simulink model "Tx_Rx"  (R2020a)
settings: Solver=VariableStepAuto  StartTime=0.0  StopTime=640e-9  RelTol=1e-3
libraries: msbUtilities x102, simulink_extras x15, dspswit3 x4, dspsigops x2
(part 2 of 3)

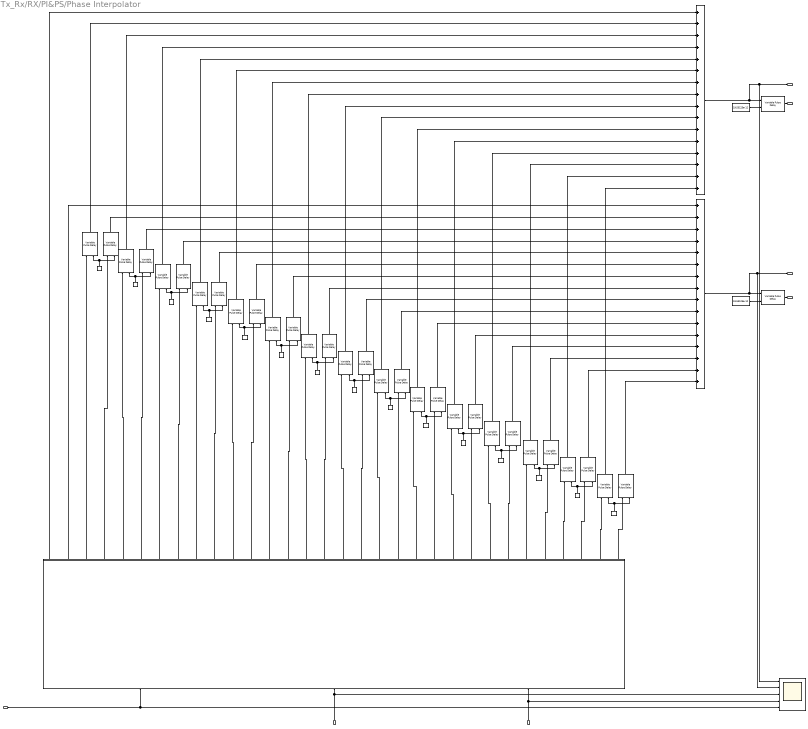
== system Tx_Rx/RX/PI&PS/Phase Interpolator ==
  CLK_s1 : Inport
  CLK_s3 : Inport  Port=2
  LSB_4bit : Inport  Port=3
  Add6 : Sum  Inputs=++++++++++++++++
  Add7 : Sum  Inputs=++++++++++++++++
  Constant26 : Constant  Value=19.53125e-12
  Constant27 : Constant  Value=0.6103515625e-12
  Constant28 : Constant  Value=2*0.6103515625e-12
  Constant29 : Constant  Value=3*0.6103515625e-12
  Constant30 : Constant  Value=4*0.6103515625e-12
  Constant31 : Constant  Value=5*0.6103515625e-12
  Constant32 : Constant  Value=6*0.6103515625e-12
  Constant33 : Constant  Value=7*0.6103515625e-12
  Constant34 : Constant  Value=8*0.6103515625e-12
  Constant35 : Constant  Value=9*0.6103515625e-12
  Constant36 : Constant  Value=10*0.6103515625e-12
  Constant37 : Constant  Value=11*0.6103515625e-12
  Constant38 : Constant  Value=12*0.6103515625e-12
  Constant39 : Constant  Value=13*0.6103515625e-12
  Constant40 : Constant  Value=14*0.6103515625e-12
  Constant41 : Constant  Value=15*0.6103515625e-12
  Constant42 : Constant  Value=19.53125e-12
  MATLAB Function : MATLAB Function  TreatAsAtomicUnit=on
  Scope : Scope  NumInputPorts=5
  Variable Pulse Delay{,1..31} (32 alike) : msbUtilities/Variable Pulse Delay  InitialInput=0  BufferSize=100
      settings: SourceProductBaseCode=AM
  CLK1 : Outport
  CLK2 : Outport  Port=2
  CLK3 : Outport  Port=3
  CLK4 : Outport  Port=4
  wires:
  Variable Pulse Delay30/1 -> Add6/16
  Constant40/1 -> Variable Pulse Delay28/2, Variable Pulse Delay29/2
  MATLAB Function/14(c6_1) -> Variable Pulse Delay13/1
  MATLAB Function/23(c11_0) -> Variable Pulse Delay22/1
  Constant34/1 -> Variable Pulse Delay17/2, Variable Pulse Delay16/2
  Constant41/1 -> Variable Pulse Delay31/2, Variable Pulse Delay30/2
  MATLAB Function/9(c4_0) -> Variable Pulse Delay8/1
  Variable Pulse Delay19/1 -> Add7/10
  Variable Pulse Delay6/1 -> Add6/4
  Constant35/1 -> Variable Pulse Delay19/2, Variable Pulse Delay18/2
  Constant27/1 -> Variable Pulse Delay2/2, Variable Pulse Delay3/2
  Variable Pulse Delay10/1 -> Add6/6
  Variable Pulse Delay25/1 -> Add7/13
  MATLAB Function/32(c15_1) -> Variable Pulse Delay31/1
  MATLAB Function/25(c12_0) -> Variable Pulse Delay24/1
  MATLAB Function/22(c10_1) -> Variable Pulse Delay21/1
  Constant33/1 -> Variable Pulse Delay15/2, Variable Pulse Delay14/2
  MATLAB Function/29(c14_0) -> Variable Pulse Delay28/1
  Constant36/1 -> Variable Pulse Delay21/2, Variable Pulse Delay20/2
  MATLAB Function/26(c12_1) -> Variable Pulse Delay25/1
  Variable Pulse Delay12/1 -> Add6/7
  Variable Pulse Delay22/1 -> Add6/12
  MATLAB Function/3(c1_0) -> Variable Pulse Delay2/1
  Constant28/1 -> Variable Pulse Delay5/2, Variable Pulse Delay4/2
  Constant31/1 -> Variable Pulse Delay11/2, Variable Pulse Delay10/2
  MATLAB Function/1(c0_0) -> Add6/1
  Constant30/1 -> Variable Pulse Delay9/2, Variable Pulse Delay8/2
  MATLAB Function/31(c15_0) -> Variable Pulse Delay30/1
  Constant38/1 -> Variable Pulse Delay25/2, Variable Pulse Delay24/2
  MATLAB Function/6(c2_1) -> Variable Pulse Delay5/1
  MATLAB Function/12(c5_1) -> Variable Pulse Delay11/1
  Variable Pulse Delay24/1 -> Add6/13
  Constant32/1 -> Variable Pulse Delay13/2, Variable Pulse Delay12/2
  MATLAB Function/17(c8_0) -> Variable Pulse Delay16/1
  MATLAB Function/15(c7_0) -> Variable Pulse Delay14/1
  Variable Pulse Delay8/1 -> Add6/5
  MATLAB Function/10(c4_1) -> Variable Pulse Delay9/1
  MATLAB Function/21(c10_0) -> Variable Pulse Delay20/1
  MATLAB Function/18(c8_1) -> Variable Pulse Delay17/1
  MATLAB Function/27(c13_0) -> Variable Pulse Delay26/1
  Variable Pulse Delay2/1 -> Add6/2
  Constant39/1 -> Variable Pulse Delay27/2, Variable Pulse Delay26/2
  MATLAB Function/2(c0_1) -> Add7/1
  Variable Pulse Delay16/1 -> Add6/9
  Variable Pulse Delay4/1 -> Add6/3
  Variable Pulse Delay18/1 -> Add6/10
  MATLAB Function/19(c9_0) -> Variable Pulse Delay18/1
  MATLAB Function/13(c6_0) -> Variable Pulse Delay12/1
  Variable Pulse Delay5/1 -> Add7/3
  Variable Pulse Delay17/1 -> Add7/9
  MATLAB Function/4(c1_1) -> Variable Pulse Delay3/1
  MATLAB Function/20(c9_1) -> Variable Pulse Delay19/1
  Variable Pulse Delay31/1 -> Add7/16
  Constant26/1 -> Variable Pulse Delay/2
  MATLAB Function/16(c7_1) -> Variable Pulse Delay15/1
  Constant42/1 -> Variable Pulse Delay1/2
  Variable Pulse Delay27/1 -> Add7/14
  Add6/1 -> CLK1/1, Scope/1, Variable Pulse Delay/1
  Variable Pulse Delay26/1 -> Add6/14
  Constant29/1 -> Variable Pulse Delay7/2, Variable Pulse Delay6/2
  Variable Pulse Delay13/1 -> Add7/7
  Variable Pulse Delay14/1 -> Add6/8
  Variable Pulse Delay29/1 -> Add7/15
  Variable Pulse Delay28/1 -> Add6/15
  MATLAB Function/28(c13_1) -> Variable Pulse Delay27/1
  Variable Pulse Delay3/1 -> Add7/2
  MATLAB Function/24(c11_1) -> Variable Pulse Delay23/1
  MATLAB Function/11(c5_0) -> Variable Pulse Delay10/1
  Variable Pulse Delay7/1 -> Add7/4
  MATLAB Function/5(c2_0) -> Variable Pulse Delay4/1
  Constant37/1 -> Variable Pulse Delay23/2, Variable Pulse Delay22/2
  MATLAB Function/30(c14_1) -> Variable Pulse Delay29/1
  Variable Pulse Delay21/1 -> Add7/11
  Variable Pulse Delay15/1 -> Add7/8
  Variable Pulse Delay20/1 -> Add6/11
  Variable Pulse Delay9/1 -> Add7/5
  Variable Pulse Delay11/1 -> Add7/6
  MATLAB Function/7(c3_0) -> Variable Pulse Delay6/1
  MATLAB Function/8(c3_1) -> Variable Pulse Delay7/1
  Variable Pulse Delay23/1 -> Add7/12
  Add7/1 -> CLK3/1, Scope/2, Variable Pulse Delay1/1
  LSB_4bit/1 -> MATLAB Function/1(LSB_4bit), Scope/5
  Variable Pulse Delay/1 -> CLK2/1
  Variable Pulse Delay1/1 -> CLK4/1
  CLK_s1/1 -> MATLAB Function/2(clk_s1), Scope/3
  CLK_s3/1 -> MATLAB Function/3(clk_s3), Scope/4

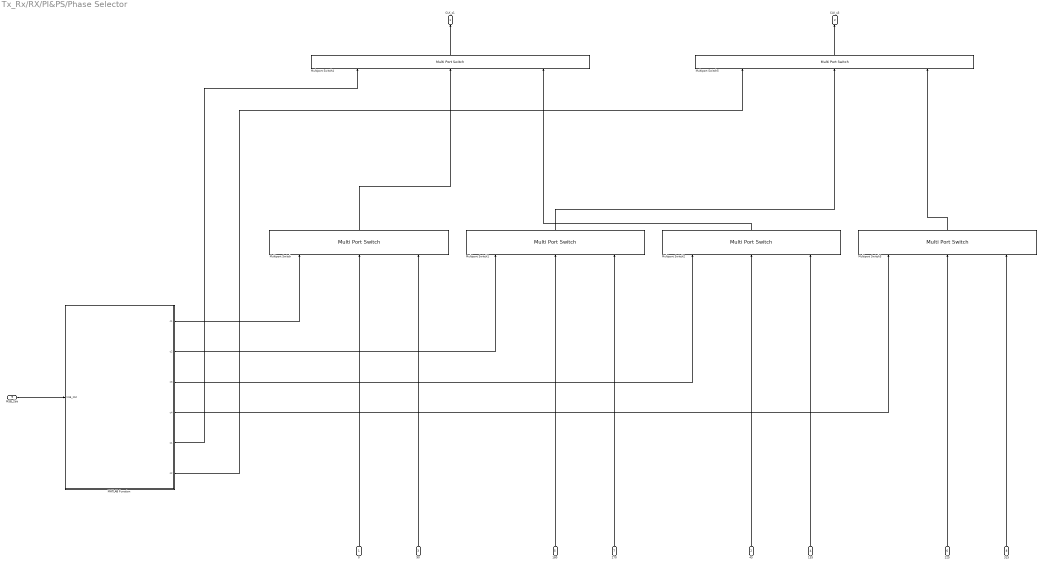
== system Tx_Rx/RX/PI&PS/Phase Selector ==
  0 : Inport
  45 : Inport  Port=2
  90 : Inport  Port=3
  135 : Inport  Port=4
  180 : Inport  Port=5
  225 : Inport  Port=6
  270 : Inport  Port=7
  315 : Inport  Port=8
  MSB_2bit : Inport  Port=9
  MATLAB Function : MATLAB Function  TreatAsAtomicUnit=on
  Multiport Switch{,1..5} (6 alike) : MultiPortSwitch  Inputs=2
  CLK_s1 : Outport
  CLK_s3 : Outport  Port=2
  wires:
  Multiport Switch1/1 -> Multiport Switch5/2
  Multiport Switch2/1 -> Multiport Switch4/3
  Multiport Switch/1 -> Multiport Switch4/2
  Multiport Switch3/1 -> Multiport Switch5/3
  225/1 -> Multiport Switch3/2
  135/1 -> Multiport Switch2/3
  0/1 -> Multiport Switch/2
  45/1 -> Multiport Switch2/2
  90/1 -> Multiport Switch/3
  315/1 -> Multiport Switch3/3
  270/1 -> Multiport Switch1/3
  180/1 -> Multiport Switch1/2
  Multiport Switch5/1 -> CLK_s3/1
  Multiport Switch4/1 -> CLK_s1/1
  MSB_2bit/1 -> MATLAB Function/1(MSB_2bit)
  MATLAB Function/1(c1) -> Multiport Switch/1
  MATLAB Function/2(c2) -> Multiport Switch1/1
  MATLAB Function/3(c3) -> Multiport Switch2/1
  MATLAB Function/4(c4) -> Multiport Switch3/1
  MATLAB Function/5(s1) -> Multiport Switch4/1
  MATLAB Function/6(s2) -> Multiport Switch5/1

== system Tx_Rx/TX/Delay Line1/Subsystem32 ==
  N-1 : Inport
  Constant : Constant
  Divide : Product  Inputs=*/
  Fref : Gain  Gain=78.125e-12
  Num : Gain  Gain=8
  Relay1 : Relay
  Variable Time Delay : VariableTransportDelay  MaximumDelay=10  FixedBuffer=on
  N : Outport
  wires:
  Num/1 -> Divide/2
  N-1/1 -> Variable Time Delay/1
  Relay1/1 -> N/1
  Divide/1 -> Fref/1
  Fref/1 -> Variable Time Delay/2
  Variable Time Delay/1 -> Relay1/1
  Constant/1 -> Num/1, Divide/1

== system Tx_Rx/TX/Delay Line1/Subsystem33 ==
  N-1 : Inport
  Constant : Constant
  Divide : Product  Inputs=*/
  Fref : Gain  Gain=78.125e-12
  Num : Gain  Gain=8
  Relay1 : Relay
  Variable Time Delay : VariableTransportDelay  MaximumDelay=10  FixedBuffer=on
  N : Outport
  wires:
  Num/1 -> Divide/2
  N-1/1 -> Variable Time Delay/1
  Relay1/1 -> N/1
  Divide/1 -> Fref/1
  Fref/1 -> Variable Time Delay/2
  Variable Time Delay/1 -> Relay1/1
  Constant/1 -> Num/1, Divide/1

== system Tx_Rx/TX/Delay Line1/Subsystem34 ==
  N-1 : Inport
  Constant : Constant
  Divide : Product  Inputs=*/
  Fref : Gain  Gain=78.125e-12
  Num : Gain  Gain=8
  Relay1 : Relay
  Variable Time Delay : VariableTransportDelay  MaximumDelay=10  FixedBuffer=on
  N : Outport
  wires:
  Num/1 -> Divide/2
  N-1/1 -> Variable Time Delay/1
  Relay1/1 -> N/1
  Divide/1 -> Fref/1
  Fref/1 -> Variable Time Delay/2
  Variable Time Delay/1 -> Relay1/1
  Constant/1 -> Num/1, Divide/1

== system Tx_Rx/TX/Delay Line1/Subsystem35 ==
  N-1 : Inport
  Constant : Constant
  Divide : Product  Inputs=*/
  Fref : Gain  Gain=78.125e-12
  Num : Gain  Gain=8
  Relay1 : Relay
  Variable Time Delay : VariableTransportDelay  MaximumDelay=10  FixedBuffer=on
  N : Outport
  wires:
  Num/1 -> Divide/2
  N-1/1 -> Variable Time Delay/1
  Relay1/1 -> N/1
  Divide/1 -> Fref/1
  Fref/1 -> Variable Time Delay/2
  Variable Time Delay/1 -> Relay1/1
  Constant/1 -> Num/1, Divide/1

== system Tx_Rx/TX/Delay Line1/Subsystem36 ==
  N-1 : Inport
  Constant : Constant
  Divide : Product  Inputs=*/
  Fref : Gain  Gain=78.125e-12
  Num : Gain  Gain=8
  Relay1 : Relay
  Variable Time Delay : VariableTransportDelay  MaximumDelay=10  FixedBuffer=on
  N : Outport
  wires:
  Num/1 -> Divide/2
  N-1/1 -> Variable Time Delay/1
  Relay1/1 -> N/1
  Divide/1 -> Fref/1
  Fref/1 -> Variable Time Delay/2
  Variable Time Delay/1 -> Relay1/1
  Constant/1 -> Num/1, Divide/1

== system Tx_Rx/TX/Delay Line1/Subsystem37 ==
  N-1 : Inport
  Constant : Constant
  Divide : Product  Inputs=*/
  Fref : Gain  Gain=78.125e-12
  Num : Gain  Gain=8
  Relay1 : Relay
  Variable Time Delay : VariableTransportDelay  MaximumDelay=10  FixedBuffer=on
  N : Outport
  wires:
  Num/1 -> Divide/2
  N-1/1 -> Variable Time Delay/1
  Relay1/1 -> N/1
  Divide/1 -> Fref/1
  Fref/1 -> Variable Time Delay/2
  Variable Time Delay/1 -> Relay1/1
  Constant/1 -> Num/1, Divide/1

== system Tx_Rx/TX/Delay Line1/Subsystem38 ==
  N-1 : Inport
  Constant : Constant
  Divide : Product  Inputs=*/
  Fref : Gain  Gain=78.125e-12
  Num : Gain  Gain=8
  Relay1 : Relay
  Variable Time Delay : VariableTransportDelay  MaximumDelay=10  FixedBuffer=on
  N : Outport
  wires:
  Num/1 -> Divide/2
  N-1/1 -> Variable Time Delay/1
  Relay1/1 -> N/1
  Divide/1 -> Fref/1
  Fref/1 -> Variable Time Delay/2
  Variable Time Delay/1 -> Relay1/1
  Constant/1 -> Num/1, Divide/1

== system Tx_Rx/TX/Delay Line1/Subsystem39 ==
  N-1 : Inport
  Constant : Constant
  Divide : Product  Inputs=*/
  Fref : Gain  Gain=78.125e-12
  Num : Gain  Gain=8
  Relay1 : Relay
  Variable Time Delay : VariableTransportDelay  MaximumDelay=10  FixedBuffer=on
  N : Outport
  wires:
  Num/1 -> Divide/2
  N-1/1 -> Variable Time Delay/1
  Relay1/1 -> N/1
  Divide/1 -> Fref/1
  Fref/1 -> Variable Time Delay/2
  Variable Time Delay/1 -> Relay1/1
  Constant/1 -> Num/1, Divide/1

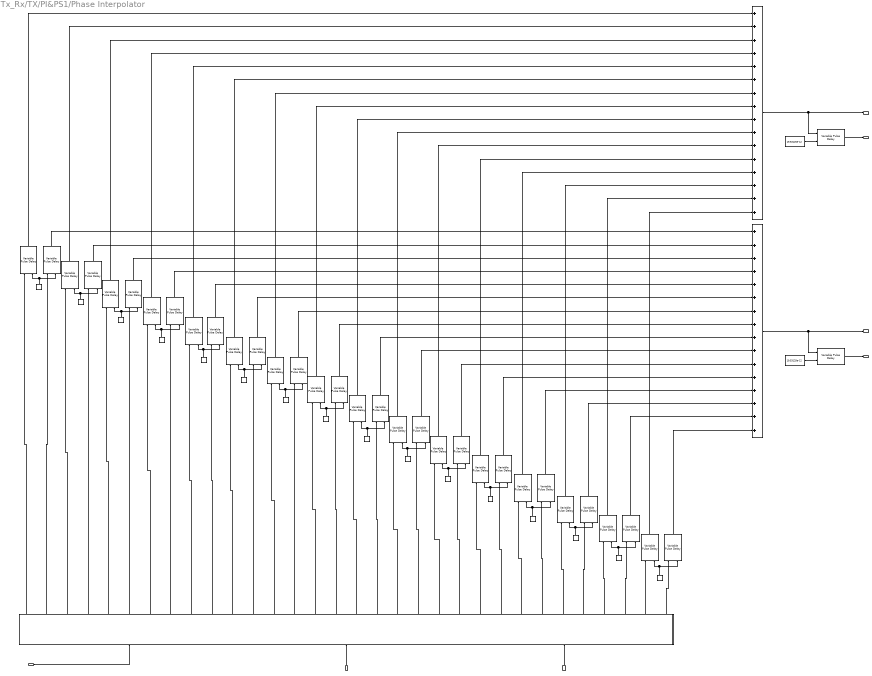
== system Tx_Rx/TX/PI&PS1/Phase Interpolator ==
  CLK_s1 : Inport
  CLK_s3 : Inport  Port=2
  LSB_4bit : Inport  Port=3
  Add6 : Sum  Inputs=++++++++++++++++
  Add7 : Sum  Inputs=++++++++++++++++
  Constant1 : Constant  Value=16*0.6103515625e-12
  Constant2 : Constant  Value=19.53125e-12
  Constant26 : Constant  Value=19.53125e-12
  Constant27 : Constant  Value=0.6103515625e-12
  Constant28 : Constant  Value=2*0.6103515625e-12
  Constant29 : Constant  Value=3*0.6103515625e-12
  Constant30 : Constant  Value=4*0.6103515625e-12
  Constant31 : Constant  Value=5*0.6103515625e-12
  Constant32 : Constant  Value=6*0.6103515625e-12
  Constant33 : Constant  Value=7*0.6103515625e-12
  Constant34 : Constant  Value=8*0.6103515625e-12
  Constant35 : Constant  Value=9*0.6103515625e-12
  Constant36 : Constant  Value=10*0.6103515625e-12
  Constant37 : Constant  Value=11*0.6103515625e-12
  Constant38 : Constant  Value=12*0.6103515625e-12
  Constant39 : Constant  Value=13*0.6103515625e-12
  Constant40 : Constant  Value=14*0.6103515625e-12
  Constant41 : Constant  Value=15*0.6103515625e-12
  MATLAB Function : MATLAB Function  TreatAsAtomicUnit=on
  Variable Pulse Delay{,1..33} (34 alike) : msbUtilities/Variable Pulse Delay  InitialInput=0  BufferSize=100
      settings: SourceProductBaseCode=AM
  CLK1 : Outport
  CLK3 : Outport  Port=2
  CLK2 : Outport  Port=3
  CLK4 : Outport  Port=4
  wires:
  Variable Pulse Delay30/1 -> Add6/16
  Constant40/1 -> Variable Pulse Delay28/2, Variable Pulse Delay29/2
  MATLAB Function/14(c6_1) -> Variable Pulse Delay13/1
  MATLAB Function/23(c11_0) -> Variable Pulse Delay22/1
  Constant34/1 -> Variable Pulse Delay17/2, Variable Pulse Delay16/2
  Constant41/1 -> Variable Pulse Delay31/2, Variable Pulse Delay30/2
  MATLAB Function/9(c4_0) -> Variable Pulse Delay8/1
  Variable Pulse Delay19/1 -> Add7/10
  Variable Pulse Delay6/1 -> Add6/4
  Constant35/1 -> Variable Pulse Delay19/2, Variable Pulse Delay18/2
  Constant27/1 -> Variable Pulse Delay2/2, Variable Pulse Delay3/2
  Variable Pulse Delay10/1 -> Add6/6
  Variable Pulse Delay25/1 -> Add7/13
  MATLAB Function/32(c15_1) -> Variable Pulse Delay31/1
  MATLAB Function/25(c12_0) -> Variable Pulse Delay24/1
  MATLAB Function/22(c10_1) -> Variable Pulse Delay21/1
  Constant33/1 -> Variable Pulse Delay15/2, Variable Pulse Delay14/2
  MATLAB Function/29(c14_0) -> Variable Pulse Delay28/1
  Constant36/1 -> Variable Pulse Delay21/2, Variable Pulse Delay20/2
  MATLAB Function/26(c12_1) -> Variable Pulse Delay25/1
  Variable Pulse Delay12/1 -> Add6/7
  Variable Pulse Delay22/1 -> Add6/12
  MATLAB Function/3(c1_0) -> Variable Pulse Delay2/1
  Constant28/1 -> Variable Pulse Delay5/2, Variable Pulse Delay4/2
  Constant31/1 -> Variable Pulse Delay11/2, Variable Pulse Delay10/2
  Constant30/1 -> Variable Pulse Delay9/2, Variable Pulse Delay8/2
  MATLAB Function/31(c15_0) -> Variable Pulse Delay30/1
  Constant38/1 -> Variable Pulse Delay25/2, Variable Pulse Delay24/2
  MATLAB Function/6(c2_1) -> Variable Pulse Delay5/1
  MATLAB Function/12(c5_1) -> Variable Pulse Delay11/1
  Variable Pulse Delay24/1 -> Add6/13
  Constant32/1 -> Variable Pulse Delay13/2, Variable Pulse Delay12/2
  MATLAB Function/17(c8_0) -> Variable Pulse Delay16/1
  MATLAB Function/15(c7_0) -> Variable Pulse Delay14/1
  Variable Pulse Delay8/1 -> Add6/5
  MATLAB Function/10(c4_1) -> Variable Pulse Delay9/1
  MATLAB Function/21(c10_0) -> Variable Pulse Delay20/1
  MATLAB Function/18(c8_1) -> Variable Pulse Delay17/1
  MATLAB Function/27(c13_0) -> Variable Pulse Delay26/1
  Variable Pulse Delay2/1 -> Add6/2
  Constant39/1 -> Variable Pulse Delay27/2, Variable Pulse Delay26/2
  Variable Pulse Delay16/1 -> Add6/9
  Variable Pulse Delay4/1 -> Add6/3
  Variable Pulse Delay18/1 -> Add6/10
  MATLAB Function/19(c9_0) -> Variable Pulse Delay18/1
  MATLAB Function/13(c6_0) -> Variable Pulse Delay12/1
  Variable Pulse Delay5/1 -> Add7/3
  Variable Pulse Delay17/1 -> Add7/9
  MATLAB Function/4(c1_1) -> Variable Pulse Delay3/1
  MATLAB Function/20(c9_1) -> Variable Pulse Delay19/1
  Variable Pulse Delay31/1 -> Add7/16
  MATLAB Function/16(c7_1) -> Variable Pulse Delay15/1
  Variable Pulse Delay27/1 -> Add7/14
  Variable Pulse Delay26/1 -> Add6/14
  Constant29/1 -> Variable Pulse Delay7/2, Variable Pulse Delay6/2
  Variable Pulse Delay13/1 -> Add7/7
  Variable Pulse Delay14/1 -> Add6/8
  Variable Pulse Delay29/1 -> Add7/15
  Variable Pulse Delay28/1 -> Add6/15
  MATLAB Function/28(c13_1) -> Variable Pulse Delay27/1
  Variable Pulse Delay3/1 -> Add7/2
  MATLAB Function/24(c11_1) -> Variable Pulse Delay23/1
  MATLAB Function/11(c5_0) -> Variable Pulse Delay10/1
  Variable Pulse Delay7/1 -> Add7/4
  MATLAB Function/5(c2_0) -> Variable Pulse Delay4/1
  Constant37/1 -> Variable Pulse Delay23/2, Variable Pulse Delay22/2
  MATLAB Function/30(c14_1) -> Variable Pulse Delay29/1
  Variable Pulse Delay21/1 -> Add7/11
  Variable Pulse Delay15/1 -> Add7/8
  Variable Pulse Delay20/1 -> Add6/11
  Variable Pulse Delay9/1 -> Add7/5
  Variable Pulse Delay11/1 -> Add7/6
  MATLAB Function/7(c3_0) -> Variable Pulse Delay6/1
  MATLAB Function/8(c3_1) -> Variable Pulse Delay7/1
  Variable Pulse Delay23/1 -> Add7/12
  LSB_4bit/1 -> MATLAB Function/1(LSB_4bit)
  Add6/1 -> Variable Pulse Delay/1, CLK1/1
  CLK_s1/1 -> MATLAB Function/2(clk_s1)
  CLK_s3/1 -> MATLAB Function/3(clk_s3)
  MATLAB Function/1(c0_0) -> Variable Pulse Delay1/1
  MATLAB Function/2(c0_1) -> Variable Pulse Delay32/1
  Variable Pulse Delay1/1 -> Add6/1
  Variable Pulse Delay32/1 -> Add7/1
  Constant1/1 -> Variable Pulse Delay32/2, Variable Pulse Delay1/2
  Variable Pulse Delay/1 -> CLK2/1
  Constant26/1 -> Variable Pulse Delay/2
  Variable Pulse Delay33/1 -> CLK4/1
  Add7/1 -> Variable Pulse Delay33/1, CLK3/1
  Constant2/1 -> Variable Pulse Delay33/2

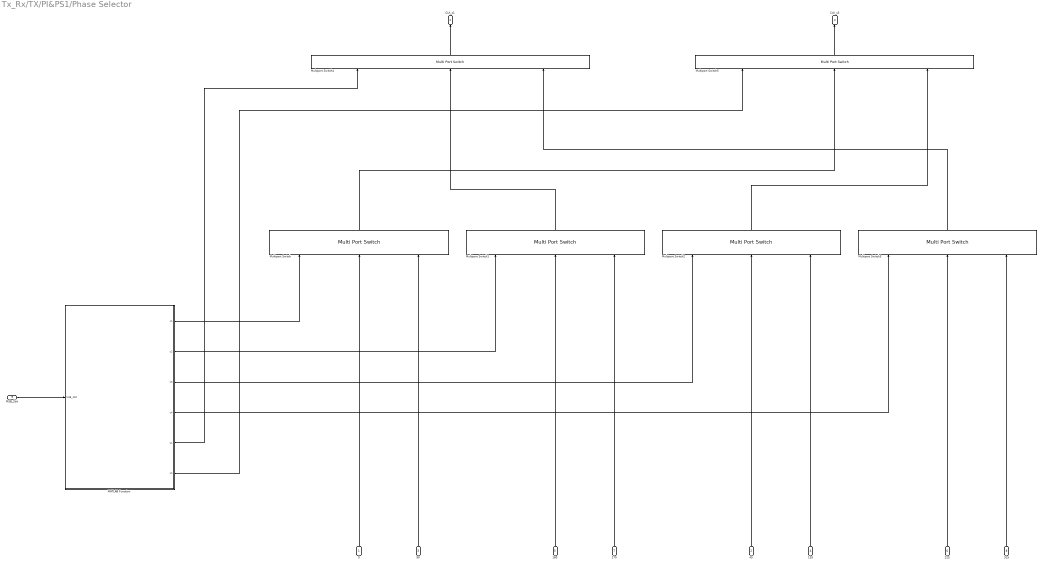
== system Tx_Rx/TX/PI&PS1/Phase Selector ==
  0 : Inport
  45 : Inport  Port=2
  90 : Inport  Port=3
  135 : Inport  Port=4
  180 : Inport  Port=5
  225 : Inport  Port=6
  270 : Inport  Port=7
  315 : Inport  Port=8
  MSB_2bit : Inport  Port=9
  MATLAB Function : MATLAB Function  TreatAsAtomicUnit=on
  Multiport Switch{,1..5} (6 alike) : MultiPortSwitch  Inputs=2
  CLK_s1 : Outport
  CLK_s3 : Outport  Port=2
  wires:
  225/1 -> Multiport Switch3/2
  135/1 -> Multiport Switch2/3
  0/1 -> Multiport Switch/2
  45/1 -> Multiport Switch2/2
  90/1 -> Multiport Switch/3
  315/1 -> Multiport Switch3/3
  270/1 -> Multiport Switch1/3
  180/1 -> Multiport Switch1/2
  Multiport Switch5/1 -> CLK_s3/1
  Multiport Switch4/1 -> CLK_s1/1
  MSB_2bit/1 -> MATLAB Function/1(MSB_2bit)
  MATLAB Function/1(c1) -> Multiport Switch/1
  MATLAB Function/2(c2) -> Multiport Switch1/1
  MATLAB Function/3(c3) -> Multiport Switch2/1
  MATLAB Function/4(c4) -> Multiport Switch3/1
  MATLAB Function/5(s1) -> Multiport Switch4/1
  MATLAB Function/6(s2) -> Multiport Switch5/1
  Multiport Switch/1 -> Multiport Switch5/2
  Multiport Switch2/1 -> Multiport Switch5/3
  Multiport Switch1/1 -> Multiport Switch4/2
  Multiport Switch3/1 -> Multiport Switch4/3

== matlab function Tx_Rx/BER_calculator/PI&PS/Phase Selector/MATLAB Function ==
  data: MSB_2bit input; c1 output; c2 output; c3 output; c4 output; s1 output; s2 output
function [c1,c2,c3,c4,s1,s2] =  bit_decoder(MSB_2bit)
    if (MSB_2bit == 0)
        c1 = 1;
        c2 = 1;
        c3 = 1;
        c4 = 1;
        s1 = 1;
        s2 = 1;
    elseif (MSB_2bit == 1)
        c1 = 2;
        c2 = 2;
        c3 = 1;
        c4 = 1;
        s1 = 2;
        s2 = 2;
    elseif (MSB_2bit == 10)
        c1 = 2;
        c2 = 2;
        c3 = 2;
        c4 = 2;
        s1 = 1;
        s2 = 1;
    elseif (MSB_2bit == 11)
        c1 = 1;
        c2 = 1;
        c3 = 2;
        c4 = 2;
        s1 = 2;
        s2 = 2;
    else
        c1 = 1;
        c2 = 1;
        c3 = 1;
        c4 = 1;
        s1 = 1;
        s2 = 1;
    end

== matlab function Tx_Rx/TX/MATLAB Function ==
  data: data_in_ref input; data_in_change input; LSB_4bit input; data_out output; MSB_2bit input
function data_out  = bypass_000000(data_in_ref,data_in_change,LSB_4bit,MSB_2bit)
    if(LSB_4bit == 0000&&MSB_2bit == 00)
        data_out = data_in_ref;
    else
        data_out = data_in_change;
    end
end

== matlab function Tx_Rx/TX/PI&PS1/Phase Interpolator/MATLAB Function ==
  data: LSB_4bit input; c0_0 output; clk_s1 input; clk_s3 input; c0_1 output; c1_0 output; c1_1 output; c2_0 output; c2_1 output; c3_0 output; c3_1 output; c4_0 output; c4_1 output; c5_0 output; c5_1 output; c6_0 output; c6_1 output; c7_0 output; c7_1 output; c8_0 output; c8_1 output; c9_0 output; c9_1 output; c10_0 output; c10_1 output; c11_0 output; c11_1 output; c12_0 output; c12_1 output; c13_0 output; c13_1 output; c14_0 output; c14_1 output; c15_0 output; c15_1 output
function [c0_0,c0_1,c1_0,c1_1,c2_0,c2_1,c3_0,c3_1,c4_0,c4_1,c5_0,c5_1,c6_0,c6_1,c7_0,c7_1,c8_0,c8_1,c9_0,c9_1,c10_0,c10_1,c11_0,c11_1,c12_0,c12_1,c13_0,c13_1,c14_0,c14_1,c15_0,c15_1] = phase_interpolator(LSB_4bit,clk_s1,clk_s3)
    switch LSB_4bit
        case 0
            c0_0 = clk_s1;
            c0_1 = clk_s3;
            c1_0 = 0;
            c1_1 = 0;
            c2_0 = 0;
            c2_1 = 0;
            c3_0 = 0;
            c3_1 = 0;
            c4_0 = 0;
            c4_1 = 0;
            c5_0 = 0;
            c5_1 = 0;
            c6_0 = 0;
            c6_1 = 0;
            c7_0 = 0;
            c7_1 = 0;
            c8_0 = 0;
            c8_1 = 0;
            c9_0 = 0;
            c9_1 = 0;
            c10_0 = 0;
            c10_1 = 0;
            c11_0 = 0;
            c11_1 = 0;
            c12_0 = 0;
            c12_1 = 0;
            c13_0 = 0;
            c13_1 = 0;
            c14_0 = 0;
            c14_1 = 0;
            c15_0 = 0;
            c15_1 = 0;
        case 1111
            c0_0 = 0;
            c0_1 = 0;
            c1_0 = clk_s1;
            c1_1 = clk_s3;
            c2_0 = 0;
            c2_1 = 0;
            c3_0 = 0;
            c3_1 = 0;
            c4_0 = 0;
            c4_1 = 0;
            c5_0 = 0;
            c5_1 = 0;
            c6_0 = 0;
            c6_1 = 0;
            c7_0 = 0;
            c7_1 = 0;
            c8_0 = 0;
            c8_1 = 0;
            c9_0 = 0;
            c9_1 = 0;
            c10_0 = 0;
            c10_1 = 0;
            c11_0 = 0;
            c11_1 = 0;
            c12_0 = 0;
            c12_1 = 0;
            c13_0 = 0;
            c13_1 = 0;
            c14_0 = 0;
            c14_1 = 0;
            c15_0 = 0;
            c15_1 = 0;
        case 1110
            c0_0 = 0;
            c0_1 = 0;
            c1_0 = 0;
            c1_1 = 0;
            c2_0 = clk_s1;
            c2_1 = clk_s3;
            c3_0 = 0;
            c3_1 = 0;
            c4_0 = 0;
            c4_1 = 0;
            c5_0 = 0;
            c5_1 = 0;
            c6_0 = 0;
            c6_1 = 0;
            c7_0 = 0;
            c7_1 = 0;
            c8_0 = 0;
            c8_1 = 0;
            c9_0 = 0;
            c9_1 = 0;
            c10_0 = 0;
            c10_1 = 0;
            c11_0 = 0;
            c11_1 = 0;
            c12_0 = 0;
            c12_1 = 0;
            c13_0 = 0;
            c13_1 = 0;
            c14_0 = 0;
            c14_1 = 0;
            c15_0 = 0;
            c15_1 = 0;
        case 1101
            c0_0 = 0;
            c0_1 = 0;
            c1_0 = 0;
            c1_1 = 0;
            c2_0 = 0;
            c2_1 = 0;
            c3_0 = clk_s1;
            c3_1 = clk_s3;
            c4_0 = 0;
            c4_1 = 0;
            c5_0 = 0;
            c5_1 = 0;
            c6_0 = 0;
            c6_1 = 0;
            c7_0 = 0;
            c7_1 = 0;
            c8_0 = 0;
            c8_1 = 0;
            c9_0 = 0;
            c9_1 = 0;
            c10_0 = 0;
            c10_1 = 0;
            c11_0 = 0;
            c11_1 = 0;
            c12_0 = 0;
            c12_1 = 0;
            c13_0 = 0;
            c13_1 = 0;
            c14_0 = 0;
            c14_1 = 0;
            c15_0 = 0;
            c15_1 = 0;
        case 1100
            c0_0 = 0;
            c0_1 = 0;
            c1_0 = 0;
            c1_1 = 0;
            c2_0 = 0;
            c2_1 = 0;
            c3_0 = 0;
            c3_1 = 0;
            c4_0 = clk_s1;
            c4_1 = clk_s3;
            c5_0 = 0;
            c5_1 = 0;
            c6_0 = 0;
            c6_1 = 0;
            c7_0 = 0;
            c7_1 = 0;
            c8_0 = 0;
            c8_1 = 0;
            c9_0 = 0;
            c9_1 = 0;
            c10_0 = 0;
            c10_1 = 0;
            c11_0 = 0;
            c11_1 = 0;
            c12_0 = 0;
            c12_1 = 0;
            c13_0 = 0;
            c13_1 = 0;
            c14_0 = 0;
            c14_1 = 0;
            c15_0 = 0;
            c15_1 = 0;
        case 1011
            c0_0 = 0;
            c0_1 = 0;
            c1_0 = 0;
            c1_1 = 0;
            c2_0 = 0;
            c2_1 = 0;
            c3_0 = 0;
            c3_1 = 0;
            c4_0 = 0;
            c4_1 = 0;
            c5_0 = clk_s1;
            c5_1 = clk_s3;
            c6_0 = 0;
            c6_1 = 0;
            c7_0 = 0;
            c7_1 = 0;
            c8_0 = 0;
            c8_1 = 0;
            c9_0 = 0;
            c9_1 = 0;
            c10_0 = 0;
            c10_1 = 0;
            c11_0 = 0;
            c11_1 = 0;
            c12_0 = 0;
            c12_1 = 0;
            c13_0 = 0;
            c13_1 = 0;
            c14_0 = 0;
            c14_1 = 0;
            c15_0 = 0;
            c15_1 = 0;
        case 1010
            c0_0 = 0;
            c0_1 = 0;
            c1_0 = 0;
            c1_1 = 0;
            c2_0 = 0;
            c2_1 = 0;
            c3_0 = 0;
            c3_1 = 0;
            c4_0 = 0;
            c4_1 = 0;
            c5_0 = 0;
            c5_1 = 0;
            c6_0 = clk_s1;
            c6_1 = clk_s3;
            c7_0 = 0;
            c7_1 = 0;
            c8_0 = 0;
            c8_1 = 0;
            c9_0 = 0;
            c9_1 = 0;
            c10_0 = 0;
            c10_1 = 0;
            c11_0 = 0;
            c11_1 = 0;
            c12_0 = 0;
            c12_1 = 0;
            c13_0 = 0;
            c13_1 = 0;
            c14_0 = 0;
            c14_1 = 0;
            c15_0 = 0;
            c15_1 = 0;
        case 1001
            c0_0 = 0;
            c0_1 = 0;
            c1_0 = 0;
            c1_1 = 0;
            c2_0 = 0;
            c2_1 = 0;
            c3_0 = 0;
            c3_1 = 0;
            c4_0 = 0;
            c4_1 = 0;
            c5_0 = 0;
            c5_1 = 0;
            c6_0 = 0;
            c6_1 = 0;
            c7_0 = clk_s1;
            c7_1 = clk_s3;
            c8_0 = 0;
            c8_1 = 0;
            c9_0 = 0;
            c9_1 = 0;
            c10_0 = 0;
            c10_1 = 0;
            c11_0 = 0;
            c11_1 = 0;
            c12_0 = 0;
            c12_1 = 0;
            c13_0 = 0;
            c13_1 = 0;
            c14_0 = 0;
            c14_1 = 0;
            c15_0 = 0;
            c15_1 = 0;
        case 1000
            c0_0 = 0;
            c0_1 = 0;
            c1_0 = 0;
            c1_1 = 0;
            c2_0 = 0;
            c2_1 = 0;
            c3_0 = 0;
            c3_1 = 0;
            c4_0 = 0;
            c4_1 = 0;
            c5_0 = 0;
            c5_1 = 0;
            c6_0 = 0;
            c6_1 = 0;
            c7_0 = 0;
            c7_1 = 0;
            c8_0 = clk_s1;
            c8_1 = clk_s3;
            c9_0 = 0;
            c9_1 = 0;
            c10_0 = 0;
            c10_1 = 0;
            c11_0 = 0;
            c11_1 = 0;
            c12_0 = 0;
            c12_1 = 0;
            c13_0 = 0;
            c13_1 = 0;
            c14_0 = 0;
            c14_1 = 0;
            c15_0 = 0;
            c15_1 = 0;
        case 111
            c0_0 = 0;
            c0_1 = 0;
            c1_0 = 0;
            c1_1 = 0;
            c2_0 = 0;
            c2_1 = 0;
            c3_0 = 0;
            c3_1 = 0;
            c4_0 = 0;
            c4_1 = 0;
            c5_0 = 0;
            c5_1 = 0;
            c6_0 = 0;
            c6_1 = 0;
            c7_0 = 0;
            c7_1 = 0;
            c8_0 = 0;
            c8_1 = 0;
            c9_0 = clk_s1;
            c9_1 = clk_s3;
            c10_0 = 0;
            c10_1 = 0;
            c11_0 = 0;
            c11_1 = 0;
            c12_0 = 0;
            c12_1 = 0;
            c13_0 = 0;
            c13_1 = 0;
            c14_0 = 0;
            c14_1 = 0;
            c15_0 = 0;
            c15_1 = 0;
        case 110
            c0_0 = 0;
            c0_1 = 0;
            c1_0 = 0;
            c1_1 = 0;
            c2_0 = 0;
            c2_1 = 0;
            c3_0 = 0;
            c3_1 = 0;
            c4_0 = 0;
            c4_1 = 0;
            c5_0 = 0;
            c5_1 = 0;
            c6_0 = 0;
            c6_1 = 0;
            c7_0 = 0;
            c7_1 = 0;
            c8_0 = 0;
            c8_1 = 0;
            c9_0 = 0;
            c9_1 = 0;
            c10_0 = clk_s1;
            c10_1 = clk_s3;
            c11_0 = 0;
            c11_1 = 0;
            c12_0 = 0;
            c12_1 = 0;
            c13_0 = 0;
            c13_1 = 0;
            c14_0 = 0;
            c14_1 = 0;
            c15_0 = 0;
            c15_1 = 0;   
        case 101
            c0_0 = 0;
            c0_1 = 0;
            c1_0 = 0;
            c1_1 = 0;
            c2_0 = 0;
            c2_1 = 0;
            c3_0 = 0;
            c3_1 = 0;
            c4_0 = 0;
            c4_1 = 0;
            c5_0 = 0;
            c5_1 = 0;
            c6_0 = 0;
            c6_1 = 0;
            c7_0 = 0;
            c7_1 = 0;
            c8_0 = 0;
            c8_1 = 0;
            c9_0 = 0;
            c9_1 = 0;
            c10_0 = 0;
            c10_1 = 0;
            c11_0 = clk_s1;
            c11_1 = clk_s3;
            c12_0 = 0;
            c12_1 = 0;
            c13_0 = 0;
            c13_1 = 0;
            c14_0 = 0;
            c14_1 = 0;
            c15_0 = 0;
            c15_1 = 0;
        case 100
            c0_0 = 0;
            c0_1 = 0;
            c1_0 = 0;
            c1_1 = 0;
            c2_0 = 0;
            c2_1 = 0;
            c3_0 = 0;
            c3_1 = 0;
            c4_0 = 0;
            c4_1 = 0;
            c5_0 = 0;
            c5_1 = 0;
            c6_0 = 0;
            c6_1 = 0;
            c7_0 = 0;
            c7_1 = 0;
            c8_0 = 0;
            c8_1 = 0;
            c9_0 = 0;
            c9_1 = 0;
            c10_0 = 0;
            c10_1 = 0;
            c11_0 = 0;
            c11_1 = 0;
            c12_0 = clk_s1;
            c12_1 = clk_s3;
            c13_0 = 0;
            c13_1 = 0;
            c14_0 = 0;
            c14_1 = 0;
            c15_0 = 0;
            c15_1 = 0;
        case 11
            c0_0 = 0;
            c0_1 = 0;
            c1_0 = 0;
            c1_1 = 0;
            c2_0 = 0;
            c2_1 = 0;
            c3_0 = 0;
            c3_1 = 0;
            c4_0 = 0;
            c4_1 = 0;
            c5_0 = 0;
            c5_1 = 0;
            c6_0 = 0;
            c6_1 = 0;
            c7_0 = 0;
            c7_1 = 0;
            c8_0 = 0;
            c8_1 = 0;
            c9_0 = 0;
            c9_1 = 0;
            c10_0 = 0;
            c10_1 = 0;
            c11_0 = 0;
            c11_1 = 0;
            c12_0 = 0;
            c12_1 = 0;
            c13_0 = clk_s1;
            c13_1 = clk_s3;
            c14_0 = 0;
            c14_1 = 0;
            c15_0 = 0;
            c15_1 = 0;
        case 10
            c0_0 = 0;
            c0_1 = 0;
            c1_0 = 0;
            c1_1 = 0;
            c2_0 = 0;
            c2_1 = 0;
            c3_0 = 0;
            c3_1 = 0;
            c4_0 = 0;
            c4_1 = 0;
            c5_0 = 0;
            c5_1 = 0;
            c6_0 = 0;
            c6_1 = 0;
            c7_0 = 0;
            c7_1 = 0;
            c8_0 = 0;
            c8_1 = 0;
            c9_0 = 0;
            c9_1 = 0;
            c10_0 = 0;
            c10_1 = 0;
            c11_0 = 0;
            c11_1 = 0;
            c12_0 = 0;
            c12_1 = 0;
            c13_0 = 0;
            c13_1 = 0;
            c14_0 = clk_s1;
            c14_1 = clk_s3;
            c15_0 = 0;
            c15_1 = 0;
        case 1
            c0_0 = 0;
            c0_1 = 0;
            c1_0 = 0;
            c1_1 = 0;
            c2_0 = 0;
            c2_1 = 0;
            c3_0 = 0;
            c3_1 = 0;
            c4_0 = 0;
            c4_1 = 0;
            c5_0 = 0;
            c5_1 = 0;
            c6_0 = 0;
            c6_1 = 0;
            c7_0 = 0;
            c7_1 = 0;
            c8_0 = 0;
            c8_1 = 0;
            c9_0 = 0;
            c9_1 = 0;
            c10_0 = 0;
            c10_1 = 0;
            c11_0 = 0;
            c11_1 = 0;
            c12_0 = 0;
            c12_1 = 0;
            c13_0 = 0;
            c13_1 = 0;
            c14_0 = 0;
            c14_1 = 0;
            c15_0 = clk_s1;
            c15_1 = clk_s3;
        otherwise
            c0_0 = 0;
            c0_1 = 0;
            c1_0 = 0;
            c1_1 = 0;
            c2_0 = 0;
            c2_1 = 0;
            c3_0 = 0;
            c3_1 = 0;
            c4_0 = 0;
            c4_1 = 0;
            c5_0 = 0;
            c5_1 = 0;
            c6_0 = 0;
            c6_1 = 0;
            c7_0 = 0;
            c7_1 = 0;
            c8_0 = 0;
            c8_1 = 0;
            c9_0 = 0;
            c9_1 = 0;
            c10_0 = 0;
            c10_1 = 0;
            c11_0 = 0;
            c11_1 = 0;
            c12_0 = 0;
            c12_1 = 0;
            c13_0 = 0;
            c13_1 = 0;
            c14_0 = 0;
            c14_1 = 0;
            c15_0 = clk_s1;
            c15_1 = clk_s3;
    end

== matlab function Tx_Rx/TX/PI&PS1/Phase Selector/MATLAB Function ==
  data: MSB_2bit input; c1 output; c2 output; c3 output; c4 output; s1 output; s2 output
function [c1,c2,c3,c4,s1,s2] =  bit_decoder(MSB_2bit)
    if (MSB_2bit == 0)
        c1 = 1;
        c2 = 1;
        c3 = 2;
        c4 = 2;
        s1 = 2;
        s2 = 2;
    elseif (MSB_2bit == 1)
        c1 = 2;
        c2 = 2;
        c3 = 1;
        c4 = 1;
        s1 = 1;
        s2 = 1;
    elseif (MSB_2bit == 10)
        c1 = 2;
        c2 = 2;
        c3 = 1;
        c4 = 1;
        s1 = 2;
        s2 = 2;
    elseif (MSB_2bit == 11)
        c1 = 1;
        c2 = 1;
        c3 = 2;
        c4 = 2;
        s1 = 1;
        s2 = 1;
    else
        c1 = 1;
        c2 = 1;
        c3 = 2;
        c4 = 2;
        s1 = 2;
        s2 = 2;
    end

== matlab function Tx_Rx/TX/De Bruijn序列生成器/MATLAB Function ==
  data: DB_seq_s output; DB_seq_p input; DB_seq_p output
function [DB_seq_s,DB_seq_p] = fcn(DB_seq_p)
    DB_seq_s = DB_seq_p(16);
    DB_seq_p = circshift(DB_seq_p',1)';
end

== matlab function Tx_Rx/RX/Binary_divider ==
  data: DATA input; MSB_2bit output; LSB_4bit output
function [MSB_2bit,LSB_4bit] = binary_divider(DATA)
    MSB_2bit_m = bitget(DATA,6:-1:5);
    LSB_4bit_m = bitget(DATA,4:-1:1);
    MSB_2bit = MSB_2bit_m(1) * 10 + MSB_2bit_m(2);
    LSB_4bit = LSB_4bit_m(1) * 1000 + LSB_4bit_m(2) * 100 + LSB_4bit_m(3) * 10 + LSB_4bit_m(4);

== stateflow chart Tx_Rx/RX/FSM ==
  state No_Shift
    entry:
    DATA = DATA;
  state CLK_Shift_left
    (default) -> (junction 45) : {DATA = DATA - 1;}
    (junction 45) -> (junction 46) [order 1] : [DATA < 0]
    (junction 45) -> (junction 47) [order 2] : {DATA = DATA;}
    (junction 46) -> (junction 48) : {DATA = 63;}
    (junction 48) -> (junction 47)
    (junction 47) -> (junction 49)
  state CLK_Shift_right
    (default) -> (junction 32) : {DATA = DATA + 1;}
    (junction 32) -> (junction 33) [order 1] : [DATA > 63]
    (junction 32) -> (junction 34) [order 2] : {DATA = DATA;}
    (junction 33) -> (junction 35) : {DATA = 0;}
    (junction 35) -> (junction 34)
    (junction 34) -> (junction 36)
  No_Shift -> No_Shift [order 3] : [E == 1]
  (default) -> No_Shift
  CLK_Shift_left -> No_Shift [order 1] : [E == 1]
  No_Shift -> CLK_Shift_left [order 2] : [E == 0 && S == 0]
  CLK_Shift_right -> No_Shift [order 1] : [E == 1]
  No_Shift -> CLK_Shift_right [order 1] : [E == 0 && S ==1]
  CLK_Shift_left -> CLK_Shift_right [order 2] : [E == 0 && S == 1]
  CLK_Shift_left -> CLK_Shift_left [order 3] : [E == 0 && S == 0]
  CLK_Shift_right -> CLK_Shift_right [order 3] : [E == 0 && S == 1]
  CLK_Shift_right -> CLK_Shift_left [order 2] : [E == 0 && S == 0]
  data: E input; S input; DATA output =0
  events: event input RISING_EDGE_EVENT

== matlab function Tx_Rx/RX/PI&PS/Phase Interpolator/MATLAB Function ==
  data: LSB_4bit input; c0_0 output; clk_s1 input; clk_s3 input; c0_1 output; c1_0 output; c1_1 output; c2_0 output; c2_1 output; c3_0 output; c3_1 output; c4_0 output; c4_1 output; c5_0 output; c5_1 output; c6_0 output; c6_1 output; c7_0 output; c7_1 output; c8_0 output; c8_1 output; c9_0 output; c9_1 output; c10_0 output; c10_1 output; c11_0 output; c11_1 output; c12_0 output; c12_1 output; c13_0 output; c13_1 output; c14_0 output; c14_1 output; c15_0 output; c15_1 output
function [c0_0,c0_1,c1_0,c1_1,c2_0,c2_1,c3_0,c3_1,c4_0,c4_1,c5_0,c5_1,c6_0,c6_1,c7_0,c7_1,c8_0,c8_1,c9_0,c9_1,c10_0,c10_1,c11_0,c11_1,c12_0,c12_1,c13_0,c13_1,c14_0,c14_1,c15_0,c15_1] = phase_interpolator(LSB_4bit,clk_s1,clk_s3)
    switch LSB_4bit
        case 0
            c0_0 = clk_s1;
            c0_1 = clk_s3;
            c1_0 = 0;
            c1_1 = 0;
            c2_0 = 0;
            c2_1 = 0;
            c3_0 = 0;
            c3_1 = 0;
            c4_0 = 0;
            c4_1 = 0;
            c5_0 = 0;
            c5_1 = 0;
            c6_0 = 0;
            c6_1 = 0;
            c7_0 = 0;
            c7_1 = 0;
            c8_0 = 0;
            c8_1 = 0;
            c9_0 = 0;
            c9_1 = 0;
            c10_0 = 0;
            c10_1 = 0;
            c11_0 = 0;
            c11_1 = 0;
            c12_0 = 0;
            c12_1 = 0;
            c13_0 = 0;
            c13_1 = 0;
            c14_0 = 0;
            c14_1 = 0;
            c15_0 = 0;
            c15_1 = 0;
        case 1
            c0_0 = 0;
            c0_1 = 0;
            c1_0 = clk_s1;
            c1_1 = clk_s3;
            c2_0 = 0;
            c2_1 = 0;
            c3_0 = 0;
            c3_1 = 0;
            c4_0 = 0;
            c4_1 = 0;
            c5_0 = 0;
            c5_1 = 0;
            c6_0 = 0;
            c6_1 = 0;
            c7_0 = 0;
            c7_1 = 0;
            c8_0 = 0;
            c8_1 = 0;
            c9_0 = 0;
            c9_1 = 0;
            c10_0 = 0;
            c10_1 = 0;
            c11_0 = 0;
            c11_1 = 0;
            c12_0 = 0;
            c12_1 = 0;
            c13_0 = 0;
            c13_1 = 0;
            c14_0 = 0;
            c14_1 = 0;
            c15_0 = 0;
            c15_1 = 0;
        case 10
            c0_0 = 0;
            c0_1 = 0;
            c1_0 = 0;
            c1_1 = 0;
            c2_0 = clk_s1;
            c2_1 = clk_s3;
            c3_0 = 0;
            c3_1 = 0;
            c4_0 = 0;
            c4_1 = 0;
            c5_0 = 0;
            c5_1 = 0;
            c6_0 = 0;
            c6_1 = 0;
            c7_0 = 0;
            c7_1 = 0;
            c8_0 = 0;
            c8_1 = 0;
            c9_0 = 0;
            c9_1 = 0;
            c10_0 = 0;
            c10_1 = 0;
            c11_0 = 0;
            c11_1 = 0;
            c12_0 = 0;
            c12_1 = 0;
            c13_0 = 0;
            c13_1 = 0;
            c14_0 = 0;
            c14_1 = 0;
            c15_0 = 0;
            c15_1 = 0;
        case 11
            c0_0 = 0;
            c0_1 = 0;
            c1_0 = 0;
            c1_1 = 0;
            c2_0 = 0;
            c2_1 = 0;
            c3_0 = clk_s1;
            c3_1 = clk_s3;
            c4_0 = 0;
            c4_1 = 0;
            c5_0 = 0;
            c5_1 = 0;
            c6_0 = 0;
            c6_1 = 0;
            c7_0 = 0;
            c7_1 = 0;
            c8_0 = 0;
            c8_1 = 0;
            c9_0 = 0;
            c9_1 = 0;
            c10_0 = 0;
            c10_1 = 0;
            c11_0 = 0;
            c11_1 = 0;
            c12_0 = 0;
            c12_1 = 0;
            c13_0 = 0;
            c13_1 = 0;
            c14_0 = 0;
            c14_1 = 0;
            c15_0 = 0;
            c15_1 = 0;
        case 100
            c0_0 = 0;
            c0_1 = 0;
            c1_0 = 0;
            c1_1 = 0;
            c2_0 = 0;
            c2_1 = 0;
            c3_0 = 0;
            c3_1 = 0;
            c4_0 = clk_s1;
            c4_1 = clk_s3;
            c5_0 = 0;
            c5_1 = 0;
            c6_0 = 0;
            c6_1 = 0;
            c7_0 = 0;
            c7_1 = 0;
            c8_0 = 0;
            c8_1 = 0;
            c9_0 = 0;
            c9_1 = 0;
            c10_0 = 0;
            c10_1 = 0;
            c11_0 = 0;
            c11_1 = 0;
            c12_0 = 0;
            c12_1 = 0;
            c13_0 = 0;
            c13_1 = 0;
            c14_0 = 0;
            c14_1 = 0;
            c15_0 = 0;
            c15_1 = 0;
        case 101
            c0_0 = 0;
            c0_1 = 0;
            c1_0 = 0;
            c1_1 = 0;
            c2_0 = 0;
            c2_1 = 0;
            c3_0 = 0;
            c3_1 = 0;
            c4_0 = 0;
            c4_1 = 0;
            c5_0 = clk_s1;
            c5_1 = clk_s3;
            c6_0 = 0;
            c6_1 = 0;
            c7_0 = 0;
            c7_1 = 0;
            c8_0 = 0;
            c8_1 = 0;
            c9_0 = 0;
            c9_1 = 0;
            c10_0 = 0;
            c10_1 = 0;
            c11_0 = 0;
            c11_1 = 0;
            c12_0 = 0;
            c12_1 = 0;
            c13_0 = 0;
            c13_1 = 0;
            c14_0 = 0;
            c14_1 = 0;
            c15_0 = 0;
            c15_1 = 0;
        case 110
            c0_0 = 0;
            c0_1 = 0;
            c1_0 = 0;
            c1_1 = 0;
            c2_0 = 0;
            c2_1 = 0;
            c3_0 = 0;
            c3_1 = 0;
            c4_0 = 0;
            c4_1 = 0;
            c5_0 = 0;
            c5_1 = 0;
            c6_0 = clk_s1;
            c6_1 = clk_s3;
            c7_0 = 0;
            c7_1 = 0;
            c8_0 = 0;
            c8_1 = 0;
            c9_0 = 0;
            c9_1 = 0;
            c10_0 = 0;
            c10_1 = 0;
            c11_0 = 0;
            c11_1 = 0;
            c12_0 = 0;
            c12_1 = 0;
            c13_0 = 0;
            c13_1 = 0;
            c14_0 = 0;
            c14_1 = 0;
            c15_0 = 0;
            c15_1 = 0;
        case 111
            c0_0 = 0;
            c0_1 = 0;
            c1_0 = 0;
            c1_1 = 0;
            c2_0 = 0;
            c2_1 = 0;
            c3_0 = 0;
            c3_1 = 0;
            c4_0 = 0;
            c4_1 = 0;
            c5_0 = 0;
            c5_1 = 0;
            c6_0 = 0;
            c6_1 = 0;
            c7_0 = clk_s1;
            c7_1 = clk_s3;
            c8_0 = 0;
            c8_1 = 0;
            c9_0 = 0;
            c9_1 = 0;
            c10_0 = 0;
            c10_1 = 0;
            c11_0 = 0;
            c11_1 = 0;
            c12_0 = 0;
            c12_1 = 0;
            c13_0 = 0;
            c13_1 = 0;
            c14_0 = 0;
            c14_1 = 0;
            c15_0 = 0;
            c15_1 = 0;
        case 1000
            c0_0 = 0;
            c0_1 = 0;
            c1_0 = 0;
            c1_1 = 0;
            c2_0 = 0;
            c2_1 = 0;
            c3_0 = 0;
            c3_1 = 0;
            c4_0 = 0;
            c4_1 = 0;
            c5_0 = 0;
            c5_1 = 0;
            c6_0 = 0;
            c6_1 = 0;
            c7_0 = 0;
            c7_1 = 0;
            c8_0 = clk_s1;
            c8_1 = clk_s3;
            c9_0 = 0;
            c9_1 = 0;
            c10_0 = 0;
            c10_1 = 0;
            c11_0 = 0;
            c11_1 = 0;
            c12_0 = 0;
            c12_1 = 0;
            c13_0 = 0;
            c13_1 = 0;
            c14_0 = 0;
            c14_1 = 0;
            c15_0 = 0;
            c15_1 = 0;
        case 1001
            c0_0 = 0;
            c0_1 = 0;
            c1_0 = 0;
            c1_1 = 0;
            c2_0 = 0;
            c2_1 = 0;
            c3_0 = 0;
            c3_1 = 0;
            c4_0 = 0;
            c4_1 = 0;
            c5_0 = 0;
            c5_1 = 0;
            c6_0 = 0;
            c6_1 = 0;
            c7_0 = 0;
            c7_1 = 0;
            c8_0 = 0;
            c8_1 = 0;
            c9_0 = clk_s1;
            c9_1 = clk_s3;
            c10_0 = 0;
            c10_1 = 0;
            c11_0 = 0;
            c11_1 = 0;
            c12_0 = 0;
            c12_1 = 0;
            c13_0 = 0;
            c13_1 = 0;
            c14_0 = 0;
            c14_1 = 0;
            c15_0 = 0;
            c15_1 = 0;
        case 1010
            c0_0 = 0;
            c0_1 = 0;
            c1_0 = 0;
            c1_1 = 0;
            c2_0 = 0;
            c2_1 = 0;
            c3_0 = 0;
            c3_1 = 0;
            c4_0 = 0;
            c4_1 = 0;
            c5_0 = 0;
            c5_1 = 0;
            c6_0 = 0;
            c6_1 = 0;
            c7_0 = 0;
            c7_1 = 0;
            c8_0 = 0;
            c8_1 = 0;
            c9_0 = 0;
            c9_1 = 0;
            c10_0 = clk_s1;
            c10_1 = clk_s3;
            c11_0 = 0;
            c11_1 = 0;
            c12_0 = 0;
            c12_1 = 0;
            c13_0 = 0;
            c13_1 = 0;
            c14_0 = 0;
            c14_1 = 0;
            c15_0 = 0;
            c15_1 = 0;   
        case 1011
            c0_0 = 0;
            c0_1 = 0;
            c1_0 = 0;
            c1_1 = 0;
            c2_0 = 0;
            c2_1 = 0;
            c3_0 = 0;
            c3_1 = 0;
            c4_0 = 0;
            c4_1 = 0;
            c5_0 = 0;
            c5_1 = 0;
            c6_0 = 0;
            c6_1 = 0;
            c7_0 = 0;
            c7_1 = 0;
            c8_0 = 0;
            c8_1 = 0;
            c9_0 = 0;
            c9_1 = 0;
            c10_0 = 0;
            c10_1 = 0;
            c11_0 = clk_s1;
            c11_1 = clk_s3;
            c12_0 = 0;
            c12_1 = 0;
            c13_0 = 0;
            c13_1 = 0;
            c14_0 = 0;
            c14_1 = 0;
            c15_0 = 0;
            c15_1 = 0;
        case 1100
            c0_0 = 0;
            c0_1 = 0;
            c1_0 = 0;
            c1_1 = 0;
            c2_0 = 0;
            c2_1 = 0;
            c3_0 = 0;
            c3_1 = 0;
            c4_0 = 0;
            c4_1 = 0;
            c5_0 = 0;
            c5_1 = 0;
            c6_0 = 0;
            c6_1 = 0;
            c7_0 = 0;
            c7_1 = 0;
            c8_0 = 0;
            c8_1 = 0;
            c9_0 = 0;
            c9_1 = 0;
            c10_0 = 0;
            c10_1 = 0;
            c11_0 = 0;
            c11_1 = 0;
            c12_0 = clk_s1;
            c12_1 = clk_s3;
            c13_0 = 0;
            c13_1 = 0;
            c14_0 = 0;
            c14_1 = 0;
            c15_0 = 0;
            c15_1 = 0;
        case 1101
            c0_0 = 0;
            c0_1 = 0;
            c1_0 = 0;
            c1_1 = 0;
            c2_0 = 0;
            c2_1 = 0;
            c3_0 = 0;
            c3_1 = 0;
            c4_0 = 0;
            c4_1 = 0;
            c5_0 = 0;
            c5_1 = 0;
            c6_0 = 0;
            c6_1 = 0;
            c7_0 = 0;
            c7_1 = 0;
            c8_0 = 0;
            c8_1 = 0;
            c9_0 = 0;
            c9_1 = 0;
            c10_0 = 0;
            c10_1 = 0;
            c11_0 = 0;
            c11_1 = 0;
            c12_0 = 0;
            c12_1 = 0;
            c13_0 = clk_s1;
            c13_1 = clk_s3;
            c14_0 = 0;
            c14_1 = 0;
            c15_0 = 0;
            c15_1 = 0;
        case 1110
            c0_0 = 0;
            c0_1 = 0;
            c1_0 = 0;
            c1_1 = 0;
            c2_0 = 0;
            c2_1 = 0;
            c3_0 = 0;
            c3_1 = 0;
            c4_0 = 0;
            c4_1 = 0;
            c5_0 = 0;
            c5_1 = 0;
            c6_0 = 0;
            c6_1 = 0;
            c7_0 = 0;
            c7_1 = 0;
            c8_0 = 0;
            c8_1 = 0;
            c9_0 = 0;
            c9_1 = 0;
            c10_0 = 0;
            c10_1 = 0;
            c11_0 = 0;
            c11_1 = 0;
            c12_0 = 0;
            c12_1 = 0;
            c13_0 = 0;
            c13_1 = 0;
            c14_0 = clk_s1;
            c14_1 = clk_s3;
            c15_0 = 0;
            c15_1 = 0;
        otherwise
            c0_0 = 0;
            c0_1 = 0;
            c1_0 = 0;
            c1_1 = 0;
            c2_0 = 0;
            c2_1 = 0;
            c3_0 = 0;
            c3_1 = 0;
            c4_0 = 0;
            c4_1 = 0;
            c5_0 = 0;
            c5_1 = 0;
            c6_0 = 0;
            c6_1 = 0;
            c7_0 = 0;
            c7_1 = 0;
            c8_0 = 0;
            c8_1 = 0;
            c9_0 = 0;
            c9_1 = 0;
            c10_0 = 0;
            c10_1 = 0;
            c11_0 = 0;
            c11_1 = 0;
            c12_0 = 0;
            c12_1 = 0;
            c13_0 = 0;
            c13_1 = 0;
            c14_0 = 0;
            c14_1 = 0;
            c15_0 = clk_s1;
            c15_1 = clk_s3;
    end

== matlab function Tx_Rx/RX/PI&PS/Phase Selector/MATLAB Function ==
  data: MSB_2bit input; c1 output; c2 output; c3 output; c4 output; s1 output; s2 output
function [c1,c2,c3,c4,s1,s2] =  bit_decoder(MSB_2bit)
    if (MSB_2bit == 0)
        c1 = 1;
        c2 = 1;
        c3 = 1;
        c4 = 1;
        s1 = 1;
        s2 = 1;
    elseif (MSB_2bit == 1)
        c1 = 2;
        c2 = 2;
        c3 = 1;
        c4 = 1;
        s1 = 2;
        s2 = 2;
    elseif (MSB_2bit == 10)
        c1 = 2;
        c2 = 2;
        c3 = 2;
        c4 = 2;
        s1 = 1;
        s2 = 1;
    elseif (MSB_2bit == 11)
        c1 = 1;
        c2 = 1;
        c3 = 2;
        c4 = 2;
        s1 = 2;
        s2 = 2;
    else
        c1 = 1;
        c2 = 1;
        c3 = 1;
        c4 = 1;
        s1 = 1;
        s2 = 1;
    end

== matlab function Tx_Rx/TX/ De Bruijn序列生成器/MATLAB Function ==
  data: DB_seq_s output; DB_seq_p input; DB_seq_p output
function [DB_seq_s,DB_seq_p] = fcn(DB_seq_p)
    DB_seq_s = DB_seq_p(16);
    DB_seq_p = circshift(DB_seq_p',1)';
end
